simulink model "DeadBlock1_export"  (Simulink 7.9)
settings: Solver=FixedStepDiscrete  StartTime=0.0  StopTime=1000000000.0  FixedStep=1  RelTol=1e-3
settings Model: Creator=boakes  LastModifiedBy=boakes
settings OptimizationCC: InlineParams=on  InlineInvariantSignals=on  EnhancedBackFolding=on
settings RTWCC: GenCodeOnly=on

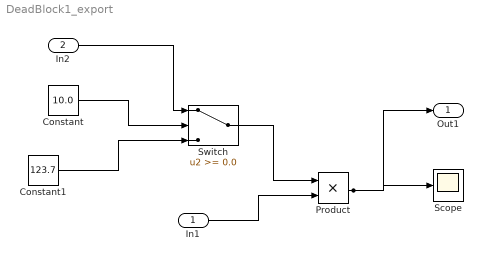
== system DeadBlock1_export ==
  In1 : Inport
  In2 : Inport  Port=2
  Constant : Constant  Value=10.0
  Constant1 : Constant  Value=123.7
  Product : Product  RndMeth=Zero
  Scope : Scope
      settings: SaveName=ScopeData2
  Switch : Switch  Threshold=0.0
  Out1 : Outport
  wires:
  Product/1 -> Scope/1, Out1/1
  Constant/1 -> Switch/2
  In1/1 -> Product/2
  In2/1 -> Switch/1
  Switch/1 -> Product/1
  Constant1/1 -> Switch/3
